simulink model "LFC_isolated_area_PI_controller"  (R2014a)
settings: Solver=ode45  StartTime=0.0  StopTime=50  RelTol=1e-3
libraries: cstblocks x10
settings Model: Creator=Divya M  LastModifiedBy=Divya M

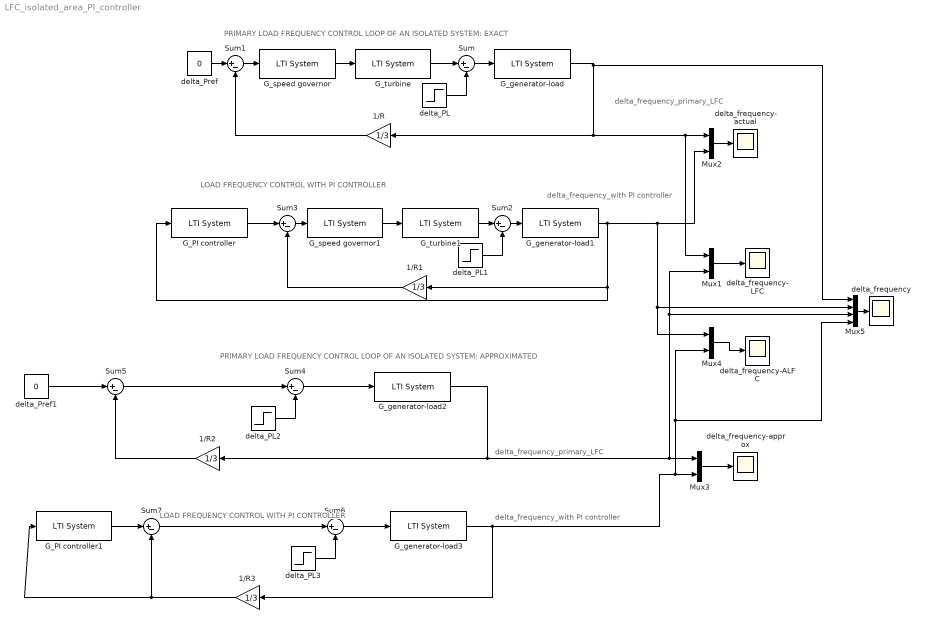
== system LFC_isolated_area_PI_controller ==
  note: PRIMARY LOAD FREQUENCY CONTROL LOOP OF AN ISOLATED SYSTEM: EXACT
  note: delta_frequency_primary_LFC
  note: LOAD FREQUENCY CONTROL WITH PI CONTROLLER
  note: delta_frequency_with PI controller
  note: PRIMARY LOAD FREQUENCY CONTROL LOOP OF AN ISOLATED SYSTEM: APPROXIMATED
  note: delta_frequency_primary_LFC
  note: LOAD FREQUENCY CONTROL WITH PI CONTROLLER
  note: delta_frequency_with PI controller
  1/R{,1..3} (4 alike) : Gain  Gain=1/3
  G_PI controller : cstblocks/LTI System  sys=tf(-.03,[1 0])  IC=[]
  G_PI controller1 : cstblocks/LTI System  sys=tf(-0.09,[1 0])  IC=[]
  G_generator-load{,1..3} (4 alike) : cstblocks/LTI System  sys=tf(100,[20 1])  IC=[]
  G_speed governor : cstblocks/LTI System  sys=tf(10,[0.4 1])  IC=[]
  G_speed governor1 : cstblocks/LTI System  sys=tf(10,[0.4 1])  IC=[]
  G_turbine : cstblocks/LTI System  sys=tf(0.1,[0.5 1])  IC=[]
  G_turbine1 : cstblocks/LTI System  sys=tf(0.1,[0.5 1])  IC=[]
  Mux{1..4} (4 alike) : Mux  Inputs=2
  Mux5 : Mux
  Sum{,1..7} (8 alike) : Sum  Inputs=|+-
  delta_PL{,1..3} (4 alike) : Step  After=0.01  SampleTime=0
  delta_Pref : Constant  Value=0
  delta_Pref1 : Constant  Value=0
  delta_frequency : Scope
      settings: YMin=-0.05  YMax=0.005  SaveName=ScopeData4
  delta_frequency- LFC : Scope
      settings: YMin=-0.05  YMax=0.005  SaveName=ScopeData3
  delta_frequency- actual : Scope
      settings: YMin=-0.05  YMax=0.005
  delta_frequency-ALFC : Scope
      settings: YMin=-0.05  YMax=0.005
  delta_frequency-approx : Scope
      settings: YMin=-0.05  YMax=0.005  SaveName=ScopeData2
  wires:
  delta_Pref/1 -> Sum1/1
  Sum1/1 -> G_speed governor/1
  G_speed governor/1 -> G_turbine/1
  G_turbine/1 -> Sum/1
  Sum/1 -> G_generator-load/1
  G_generator-load/1 -> Mux5/1, Mux1/1, Mux2/1, 1/R/1
  delta_PL/1 -> Sum/2
  1/R/1 -> Sum1/2
  Sum3/1 -> G_speed governor1/1
  G_speed governor1/1 -> G_turbine1/1
  G_turbine1/1 -> Sum2/1
  Sum2/1 -> G_generator-load1/1
  G_generator-load1/1 -> Mux5/2, Mux4/1, Mux2/2, G_PI controller/1, 1/R1/1
  delta_PL1/1 -> Sum2/2
  1/R1/1 -> Sum3/2
  G_PI controller/1 -> Sum3/1
  delta_Pref1/1 -> Sum5/1
  Sum4/1 -> G_generator-load2/1
  G_generator-load2/1 -> Mux5/3, Mux1/2, Mux3/1, 1/R2/1
  delta_PL2/1 -> Sum4/2
  1/R2/1 -> Sum5/2
  Sum7/1 -> Sum6/1
  Sum6/1 -> G_generator-load3/1
  G_generator-load3/1 -> 1/R3/1, Mux4/2, Mux5/4, Mux3/2
  delta_PL3/1 -> Sum6/2
  1/R3/1 -> G_PI controller1/1, Sum7/2
  G_PI controller1/1 -> Sum7/1
  Sum5/1 -> Sum4/1
  Mux2/1 -> delta_frequency- actual/1
  Mux3/1 -> delta_frequency-approx/1
  Mux1/1 -> delta_frequency- LFC/1
  Mux4/1 -> delta_frequency-ALFC/1
  Mux5/1 -> delta_frequency/1
